simulink model "SMO_PLL_dq_model"  (R2024b)
settings: Solver=ode23  StartTime=0.0  StopTime=0.25  FixedStep=2e-7  RelTol=1e-3
InitFcn:
  | pn = 3;
  | Ld = 1.6e-3;
  | Lq = 1e-3;
  | Ls = Ld;
  | R = 0.011;
  | phi = 0.077;
  | J = 0.0008;
  | B = 0.000;
  | Ts = 1e-5;
undefined symbols (not defined in the file or in its folder): DiscIntNeverNeededParam
libraries: spsGroundLib x1, spsUniversalBridgeLib x1, spsPermanentMagnetSynchronousMachineLib x1, spsSVPWMGenerator2LevelLib x1, spsDCVoltageSourceLib x1, spspowerguiLib x1

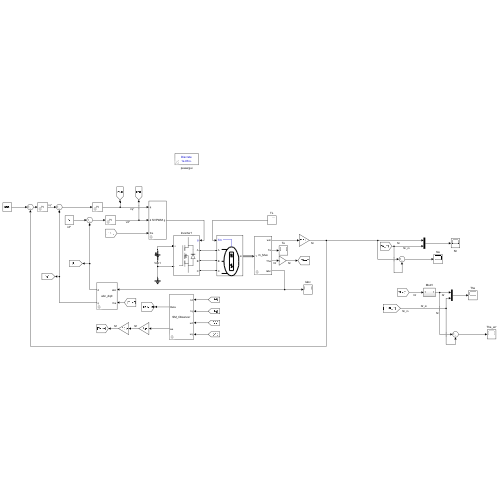
[thumbnail: Simulink's stored preview of the top-level diagram]
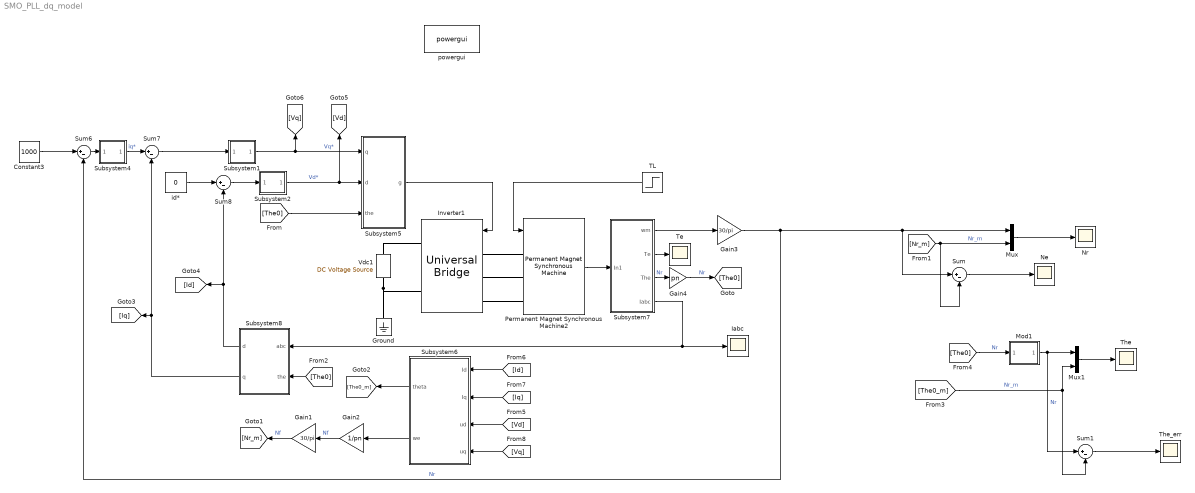
== system SMO_PLL_dq_model ==
  Constant3 : Constant  Value=1000
  Gain1 : Gain  Gain=30/pi
  Gain2 : Gain  Gain=1/pn
  Gain3 : Gain  Gain=30/pi
  Gain4 : Gain  Gain=pn
  Ground : spsGroundLib/Ground  LConnTagsString=a
  Iabc : Scope
  Inverter1 : spsUniversalBridgeLib/Universal Bridge  Arms=3  SnubberResistance=1e5  SnubberCapacitance=inf  Device=MOSFET / Diodes  Ron=1e-3  Lon=0  ForwardVoltages="[  0  0  ]"  ForwardVoltage=0  GTOparameters=[ 10e-6 , 20e-6 ]  IGBTparameters=[ 1e-6 , 2e-6 ]  Measurements=None  Measurements_2=None  converterType=Rectifier
  Mod1 : Subsystem
  Mux : Mux  Inputs=2
  Mux1 : Mux  Inputs=2
  Ne : Scope
  Nr : Scope
  Permanent Magnet Synchronous Machine2 : spsPermanentMagnetSynchronousMachineLib/Permanent Magnet Synchronous Machine  NbPhases=3  FluxDistribution=Sinusoidal  RotorType=Salient-pole  MechanicalLoad=Torque Tm  PresetModel=No  ShowDetailedParameters=on  MeasurementBus=off  Resistance=R  Inductance=8.5e-3  dqInductances=[Ld Lq]  La=0.000395  MachineConstant=Flux linkage established by magnets (V.s)  Flux=phi  VoltageCst=41.8988  TorqueCst=0.3465  Flat=120  Mechanical=[J B pn 0]  PolePairs=2  InitialConditions=[0,0, 0,0]  InitialConditions5ph=[0 0 0 0 0 0]  RefAngle=Aligned with phase A axis (original Park)  IterativeDiscreteModel=Trapezoidal non iterative  TsBlock=-1  TsPowergui=0
  Subsystem1 : Subsystem  mask{Ki=20000*R, Kp=20000*Lq, int_limit=[-161,161], out_limit=[-161,161], Ts=1/(10e3)}
      mask prompts: Ki "Ki : Integral"; Kp "Kp : Propotional"; int_limit "integral limit : [min, max]"; out_limit "output limit : [min, max]"; Ts "Ts : sample time"
  Subsystem2 : Subsystem  mask{Ki=10000*R, Kp=10000*Ld, int_limit=[-161,161], out_limit=[-161,161], Ts=1/(10e3)}
      mask prompts: Ki "Ki : Integral"; Kp "Kp : Propotional"; int_limit "integral limit : [min, max]"; out_limit "output limit : [min, max]"; Ts "Ts : sample time"
  Subsystem4 : Subsystem  mask{Ki=20, Kp=0.1, int_limit=[-200,200], out_limit=[-200,200], Ts=1/(5e3)}
      mask prompts: Ki "Ki : Integral"; Kp "Kp : Propotional"; int_limit "integral limit : [min, max]"; out_limit "output limit : [min, max]"; Ts "Ts : sample time"
  Subsystem5 : Subsystem  mask{Vdc=311}
  Subsystem6 : Subsystem  mask{Ts=1/(10e3), wc=300}
      mask prompts: Ts "Ts : sample time"; wc "wc : cross frequency (rad/s)"
  Subsystem7 : Subsystem
  Subsystem8 : Subsystem
  Sum{,1,6..8} (5 alike) : Sum  Inputs=|+-
  TL : Step  Time=0.1  After=10  SampleTime=0
  Te : Scope
  The : Scope
  The_err : Scope
  Vdc1 : spsDCVoltageSourceLib/DC Voltage Source  Amplitude=311  Measurements=None
  id* : Constant  Value=0
  powergui : spspowerguiLib/powergui  Priority=1  SimulationMode=Discrete  SampleTime=10e-7  frequency=60  Iterations=50  frequencyindice=0  Pbase=100e6  ErrMax=1e-4  UnitsV=kV  UnitsW=MW  buscounter=0  FunctionMessages=off  echomessages=off  EnableUseOfTLC=off  CurrentSourceSwitches=off  DisableSnubberDevices=off  DisableRonSwitches=off  DisableVfSwitches=off  DisplayEquations=off  AutomaticDiscreteSolvers=off  SolverType=Tustin/Backward Euler (TBE)  Interpol=off  ExternalGateDelay=off  methode=off  Ts=100  x0status=blocks  SPID=on  SwTol=0  HookPort=off  NonlinearTolerance=1e-4  nMaxIteration=100  ContinueOnMaxIteration=off  RestoreLinks=warning  ResistiveCurrentMeasurement=off  Frange=[0:2:500]  Ylog=off  Xlog=on  ShowGrid=off  save=off  variable=ZData  structure=0  ZoomFFT=off  StartTime=0.0  cycles=1  DisplayStyle=1  fundamental=60  FreqAxis=off  MaxFrequency=1000  frequencyindicesteady=1  RmsSteady=1  display=off
  wires:
  Sum7/1 -> Subsystem1/1(Input)
  Sum6/1 -> Subsystem4/1(Input)
  Subsystem4/1(output) -> Sum7/1  "iq*"
  Constant3/1 -> Sum6/1
  Subsystem5/1(g) -> Inverter1/1
  Subsystem7/1(wm) -> Gain3/1
  id*/1 -> Sum8/1
  Subsystem1/1(output) -> [Vq], Subsystem5/1(q)  "Vq*"
  Sum8/1 -> Subsystem2/1(Input)
  Subsystem2/1(output) -> Subsystem5/2(d), [Vd]  "Vd*"
  Subsystem8/2(q) -> [Iq], Sum7/2
  Subsystem7/2(Te) -> Te/1
  [The0] -> Subsystem5/3(the)
  Gain2/1 -> Gain1/1  "Nf"
  Subsystem6/2(we) -> Gain2/1
  Gain3/1 -> Sum6/2, Sum/1, Mux/1  "Nr"
  Mux/1 -> Nr/1
  Sum/1 -> Ne/1
  Subsystem7/3(The) -> Gain4/1  "Nr"
  TL/1 -> Permanent Magnet Synchronous Machine2/1
  Permanent Magnet Synchronous Machine2/1 -> Subsystem7/1(In1)
  [The0] -> Subsystem8/2(the)
  Gain4/1 -> [The0]  "Nr"
  Gain1/1 -> [Nr_m]  "Nf"
  [Nr_m] -> Sum/2, Mux/2  "Nr_m"
  Subsystem6/1(theta) -> [The0_m]
  [The0] -> Mod1/1(In1)  "Nr"
  Mux1/1 -> The/1
  [The0_m] -> Mux1/2, Sum1/2  "Nr_m"
  Mod1/1(Out1) -> Sum1/1, Mux1/1  "Nr"
  Sum1/1 -> The_err/1
  [Vq] -> Subsystem6/4(uq)
  [Vd] -> Subsystem6/3(ud)
  Subsystem8/1(d) -> [Id], Sum8/2
  [Id] -> Subsystem6/1(Id)
  [Iq] -> Subsystem6/2(Iq)
  Subsystem7/4(Iabc) -> Subsystem8/1(abc), Iabc/1
  connections:
  Vdc1/LConn1 -- Inverter1/RConn2 -- Ground/LConn1
  Vdc1/RConn1 -- Inverter1/RConn1
  Permanent Magnet Synchronous Machine2/LConn1 -- Inverter1/LConn1
  Inverter1/LConn3 -- Permanent Magnet Synchronous Machine2/LConn3
  Permanent Magnet Synchronous Machine2/LConn2 -- Inverter1/LConn2

== system SMO_PLL_dq_model/Mod1 ==
  In1 : Inport
  Constant1 : Constant  Value=2*pi
  Math Function : Math  Operator=mod  SignedPower=on
  Out1 : Outport
  wires:
  In1/1 -> Math Function/1
  Math Function/1 -> Out1/1
  Constant1/1 -> Math Function/2

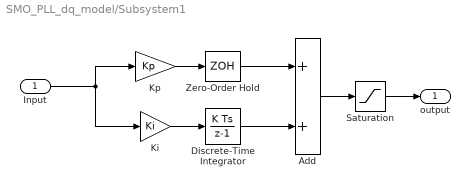
== system SMO_PLL_dq_model/Subsystem1 ==
  Input : Inport
  Add : Sum
  Discrete-Time Integrator : DiscreteIntegrator  SampleTime=Ts  LimitOutput=on  UpperSaturationLimit=int_limit(2)  LowerSaturationLimit=int_limit(1)  ICPrevOutput=DiscIntNeverNeededParam  ICPrevScaledInput=DiscIntNeverNeededParam
  Ki : Gain  Gain=Ki
  Kp : Gain  Gain=Kp
  Saturation : Saturate  UpperLimit=out_limit(2)  LowerLimit=out_limit(1)
  Zero-Order Hold : ZeroOrderHold  SampleTime=Ts
  output : Outport
  wires:
  Input/1 -> Ki/1, Kp/1
  Ki/1 -> Discrete-Time Integrator/1
  Discrete-Time Integrator/1 -> Add/2
  Add/1 -> Saturation/1
  Saturation/1 -> output/1
  Kp/1 -> Zero-Order Hold/1
  Zero-Order Hold/1 -> Add/1

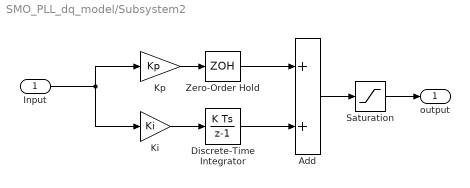
== system SMO_PLL_dq_model/Subsystem2 ==
  Input : Inport
  Add : Sum
  Discrete-Time Integrator : DiscreteIntegrator  SampleTime=Ts  LimitOutput=on  UpperSaturationLimit=int_limit(2)  LowerSaturationLimit=int_limit(1)  ICPrevOutput=DiscIntNeverNeededParam  ICPrevScaledInput=DiscIntNeverNeededParam
  Ki : Gain  Gain=Ki
  Kp : Gain  Gain=Kp
  Saturation : Saturate  UpperLimit=out_limit(2)  LowerLimit=out_limit(1)
  Zero-Order Hold : ZeroOrderHold  SampleTime=Ts
  output : Outport
  wires:
  Input/1 -> Ki/1, Kp/1
  Ki/1 -> Discrete-Time Integrator/1
  Discrete-Time Integrator/1 -> Add/2
  Add/1 -> Saturation/1
  Saturation/1 -> output/1
  Kp/1 -> Zero-Order Hold/1
  Zero-Order Hold/1 -> Add/1

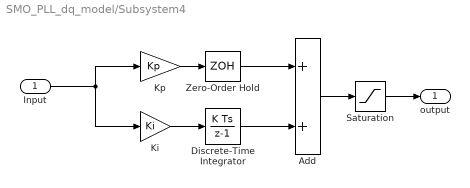
== system SMO_PLL_dq_model/Subsystem4 ==
  Input : Inport
  Add : Sum
  Discrete-Time Integrator : DiscreteIntegrator  SampleTime=Ts  LimitOutput=on  UpperSaturationLimit=int_limit(2)  LowerSaturationLimit=int_limit(1)  ICPrevOutput=DiscIntNeverNeededParam  ICPrevScaledInput=DiscIntNeverNeededParam
  Ki : Gain  Gain=Ki
  Kp : Gain  Gain=Kp
  Saturation : Saturate  UpperLimit=out_limit(2)  LowerLimit=out_limit(1)
  Zero-Order Hold : ZeroOrderHold  SampleTime=Ts
  output : Outport
  wires:
  Input/1 -> Ki/1, Kp/1
  Ki/1 -> Discrete-Time Integrator/1
  Discrete-Time Integrator/1 -> Add/2
  Add/1 -> Saturation/1
  Saturation/1 -> output/1
  Kp/1 -> Zero-Order Hold/1
  Zero-Order Hold/1 -> Add/1

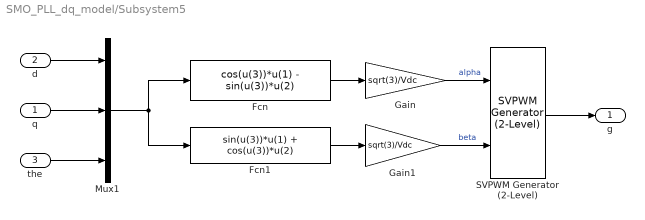
== system SMO_PLL_dq_model/Subsystem5 ==
  q : Inport
  d : Inport  Port=2
  the : Inport  Port=3
  Fcn : Fcn  Expr=cos(u(3))*u(1) - sin(u(3))*u(2)
  Fcn1 : Fcn  Expr=sin(u(3))*u(1) + cos(u(3))*u(2)
  Gain : Gain  Gain=sqrt(3)/Vdc
  Gain1 : Gain  Gain=sqrt(3)/Vdc
  Mux1 : Mux  Inputs=3
  SVPWM Generator (2-Level) : spsSVPWMGenerator2LevelLib/SVPWM Generator (2-Level)  InputType=alpha-beta components  SwitchingPattern=Pattern #1  Fc=10e3  ParUref=[0.8 -30 50]  Ts=0
  g : Outport
  wires:
  q/1 -> Mux1/2
  Fcn/1 -> Gain/1
  d/1 -> Mux1/1
  Fcn1/1 -> Gain1/1
  SVPWM Generator (2-Level)/1 -> g/1
  Mux1/1 -> Fcn/1, Fcn1/1
  the/1 -> Mux1/3
  Gain/1 -> SVPWM Generator (2-Level)/1  "alpha"
  Gain1/1 -> SVPWM Generator (2-Level)/2  "beta"

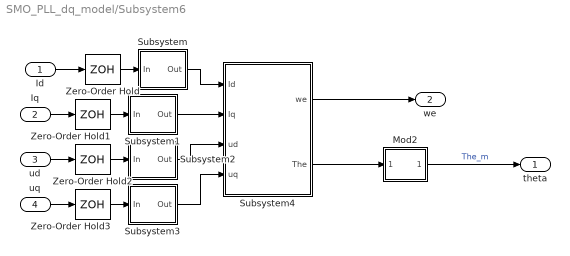
== system SMO_PLL_dq_model/Subsystem6 ==
  Id : Inport
  Iq : Inport  Port=2
  ud : Inport  Port=3
  uq : Inport  Port=4
  Mod2 : Subsystem
  Subsystem : Subsystem  mask{Ts=Ts, wc=wc}
      mask prompts: Ts "Ts ：sample time"; wc "wc : cross frequency (rad/s)"
  Subsystem1 : Subsystem  mask{Ts=Ts, wc=wc}
      mask prompts: Ts "Ts ：sample time"; wc "wc : cross frequency (rad/s)"
  Subsystem2 : Subsystem  mask{Ts=Ts, wc=wc}
      mask prompts: Ts "Ts ：sample time"; wc "wc : cross frequency (rad/s)"
  Subsystem3 : Subsystem  mask{Ts=Ts, wc=wc}
      mask prompts: Ts "Ts ：sample time"; wc "wc : cross frequency (rad/s)"
  Subsystem4 : Subsystem
  Zero-Order Hold{,1..3} (4 alike) : ZeroOrderHold  SampleTime=Ts
  theta : Outport
  we : Outport  Port=2
  wires:
  Subsystem4/1(we) -> we/1
  Subsystem4/2(The) -> Mod2/1(In1)
  Mod2/1(theta) -> theta/1  "The_m"
  Id/1 -> Zero-Order Hold/1
  Zero-Order Hold/1 -> Subsystem/1(In)
  Subsystem/1(Out) -> Subsystem4/1(Id)
  Subsystem1/1(Out) -> Subsystem4/2(Iq)
  Iq/1 -> Zero-Order Hold1/1
  Zero-Order Hold1/1 -> Subsystem1/1(In)
  Subsystem2/1(Out) -> Subsystem4/3(ud)
  ud/1 -> Zero-Order Hold2/1
  Zero-Order Hold2/1 -> Subsystem2/1(In)
  Subsystem3/1(Out) -> Subsystem4/4(uq)
  uq/1 -> Zero-Order Hold3/1
  Zero-Order Hold3/1 -> Subsystem3/1(In)

== system SMO_PLL_dq_model/Subsystem7 ==
  In1 : Inport
  Bus Selector1 : BusSelector  OutputSignals=Rotor speed wm (rad/s),Electromagnetic torque Te (N*m),Rotor angle thetam (rad),Stator current is_a (A),Stator current is_b (A),Stator current is_c (A)
  Mux : Mux  Inputs=3
  wm : Outport
  Te : Outport  Port=2
  The : Outport  Port=3
  Iabc : Outport  Port=4
  wires:
  In1/1 -> Bus Selector1/1
  Bus Selector1/1 -> wm/1  "<Rotor speed wm (rad/s)>"
  Bus Selector1/2 -> Te/1  "<Electromagnetic torque Te (N*m)>"
  Bus Selector1/3 -> The/1  "<Rotor angle thetam (rad)>"
  Bus Selector1/4 -> Mux/1  "<Stator current is_a (A)>"
  Bus Selector1/5 -> Mux/2  "<Stator current is_b (A)>"
  Bus Selector1/6 -> Mux/3  "<Stator current is_c (A)>"
  Mux/1 -> Iabc/1

== system SMO_PLL_dq_model/Subsystem8 ==
  abc : Inport
  the : Inport  Port=2
  Subsystem : Subsystem
  Subsystem5 : Subsystem
  d : Outport
  q : Outport  Port=2
  wires:
  Subsystem/1(d) -> d/1
  the/1 -> Subsystem/3(the)
  Subsystem5/2(beta) -> Subsystem/2(beta)
  Subsystem5/1(alpha) -> Subsystem/1(alpha)
  abc/1 -> Subsystem5/1(input)
  Subsystem/2(q) -> q/1

== system SMO_PLL_dq_model/Subsystem6/Mod2 ==
  In1 : Inport
  Constant1 : Constant  Value=2*pi
  Math Function : Math  Operator=mod  SignedPower=on
  theta : Outport
  wires:
  In1/1 -> Math Function/1
  Math Function/1 -> theta/1
  Constant1/1 -> Math Function/2

== system SMO_PLL_dq_model/Subsystem6/Subsystem ==
  In : Inport
  Delay : Delay  DelayLength=1  SampleTime=Ts
  Sum1 : Sum  Inputs=|++
  alpha : Gain  Gain=wc*Ts
  alpha1 : Gain  Gain=1-wc*Ts
  Out : Outport
  wires:
  alpha/1 -> Sum1/1
  Delay/1 -> alpha1/1
  In/1 -> alpha/1
  Sum1/1 -> Out/1, Delay/1
  alpha1/1 -> Sum1/2

== system SMO_PLL_dq_model/Subsystem6/Subsystem1 ==
  In : Inport
  Delay : Delay  DelayLength=1  SampleTime=Ts
  Sum1 : Sum  Inputs=|++
  alpha : Gain  Gain=wc*Ts
  alpha1 : Gain  Gain=1-wc*Ts
  Out : Outport
  wires:
  alpha/1 -> Sum1/1
  Delay/1 -> alpha1/1
  In/1 -> alpha/1
  Sum1/1 -> Out/1, Delay/1
  alpha1/1 -> Sum1/2

== system SMO_PLL_dq_model/Subsystem6/Subsystem2 ==
  In : Inport
  Delay : Delay  DelayLength=1  SampleTime=Ts
  Sum1 : Sum  Inputs=|++
  alpha : Gain  Gain=wc*Ts
  alpha1 : Gain  Gain=1-wc*Ts
  Out : Outport
  wires:
  alpha/1 -> Sum1/1
  Delay/1 -> alpha1/1
  In/1 -> alpha/1
  Sum1/1 -> Out/1, Delay/1
  alpha1/1 -> Sum1/2

== system SMO_PLL_dq_model/Subsystem6/Subsystem3 ==
  In : Inport
  Delay : Delay  DelayLength=1  SampleTime=Ts
  Sum1 : Sum  Inputs=|++
  alpha : Gain  Gain=wc*Ts
  alpha1 : Gain  Gain=1-wc*Ts
  Out : Outport
  wires:
  alpha/1 -> Sum1/1
  Delay/1 -> alpha1/1
  In/1 -> alpha/1
  Sum1/1 -> Out/1, Delay/1
  alpha1/1 -> Sum1/2

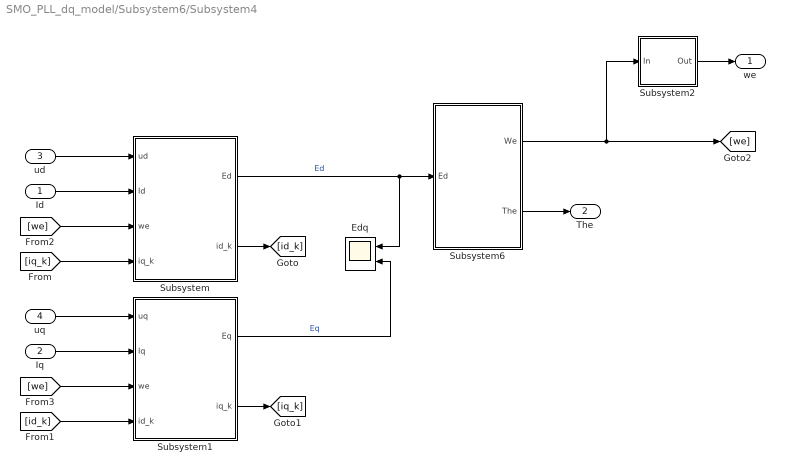
== system SMO_PLL_dq_model/Subsystem6/Subsystem4 ==
  Id : Inport
  Iq : Inport  Port=2
  ud : Inport  Port=3
  uq : Inport  Port=4
  Edq : Scope  NumInputPorts=2
  Subsystem : Subsystem
  Subsystem1 : Subsystem
  Subsystem2 : Subsystem  mask{Ts=Ts, wc=wc/3}
      mask prompts: Ts "Ts ：sample time"; wc "wc : cross frequency (rad/s)"
  Subsystem6 : Subsystem
  we : Outport
  The : Outport  Port=2
  wires:
  ud/1 -> Subsystem/1(ud)
  Id/1 -> Subsystem/2(Id)
  uq/1 -> Subsystem1/1(uq)
  Iq/1 -> Subsystem1/2(Iq)
  Subsystem/1(Ed) -> Subsystem6/1(Ed), Edq/1  "Ed"
  Subsystem1/1(Eq) -> Edq/2  "Eq"
  Subsystem/2(id_k) -> [id_k]
  Subsystem1/2(iq_k) -> [iq_k]
  [iq_k] -> Subsystem/4(iq_k)
  [id_k] -> Subsystem1/4(id_k)
  [we] -> Subsystem/3(we)
  [we] -> Subsystem1/3(we)
  Subsystem6/1(We) -> Subsystem2/1(In), [we]
  Subsystem6/2(The) -> The/1
  Subsystem2/1(Out) -> we/1

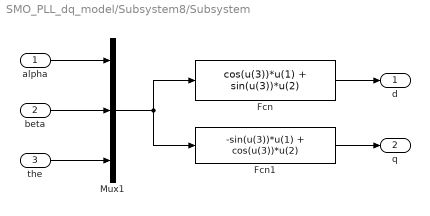
== system SMO_PLL_dq_model/Subsystem8/Subsystem ==
  alpha : Inport
  beta : Inport  Port=2
  the : Inport  Port=3
  Fcn : Fcn  Expr=cos(u(3))*u(1) + sin(u(3))*u(2)
  Fcn1 : Fcn  Expr=-sin(u(3))*u(1) + cos(u(3))*u(2)
  Mux1 : Mux  Inputs=3
  d : Outport
  q : Outport  Port=2
  wires:
  Fcn/1 -> d/1
  Mux1/1 -> Fcn/1, Fcn1/1
  the/1 -> Mux1/3
  beta/1 -> Mux1/2
  Fcn1/1 -> q/1
  alpha/1 -> Mux1/1

== system SMO_PLL_dq_model/Subsystem8/Subsystem5 ==
  input : Inport
  Demux : Demux  Outputs=3
  Subsystem : Subsystem
  alpha : Outport
  beta : Outport  Port=2
  wires:
  input/1 -> Demux/1
  Demux/1 -> Subsystem/1(a)
  Demux/2 -> Subsystem/2(b)
  Demux/3 -> Subsystem/3(c)
  Subsystem/1(alpha) -> alpha/1
  Subsystem/2(beta) -> beta/1

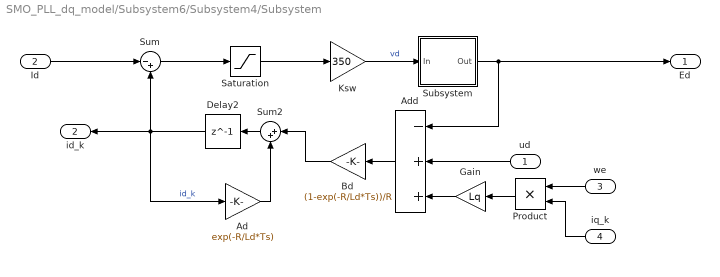
== system SMO_PLL_dq_model/Subsystem6/Subsystem4/Subsystem ==
  ud : Inport
  Id : Inport  Port=2
  we : Inport  Port=3
  iq_k : Inport  Port=4
  Ad : Gain  Gain=exp(-R/Ld*Ts)
  Add : Sum  Inputs=-++
  Bd : Gain  Gain=(1-exp(-R/Ld*Ts))/R
  Delay2 : Delay  DelayLength=1  SampleTime=Ts
  Gain : Gain  Gain=Lq
  Ksw : Gain  Gain=350
  Product : Product
  Saturation : Saturate  UpperLimit=2  LowerLimit=-2
  Subsystem : Subsystem  mask{Ts=Ts, wc=wc}
      mask prompts: Ts "Ts ：sample time"; wc "wc : cross frequency (rad/s)"
  Sum : Sum  Inputs=|-+
  Sum2 : Sum  Inputs=|++
  Ed : Outport
  id_k : Outport  Port=2
  wires:
  Ksw/1 -> Subsystem/1(In)  "vd"
  Sum/1 -> Saturation/1
  Saturation/1 -> Ksw/1
  ud/1 -> Add/2
  Add/1 -> Bd/1
  Bd/1 -> Sum2/1
  Id/1 -> Sum/1
  Ad/1 -> Sum2/2
  Delay2/1 -> id_k/1, Ad/1, Sum/2  "id_k"
  Sum2/1 -> Delay2/1
  Subsystem/1(Out) -> Add/1, Ed/1
  Gain/1 -> Add/3
  Product/1 -> Gain/1
  we/1 -> Product/1
  iq_k/1 -> Product/2

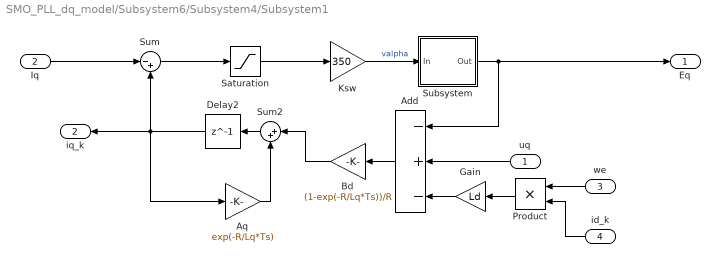
== system SMO_PLL_dq_model/Subsystem6/Subsystem4/Subsystem1 ==
  uq : Inport
  Iq : Inport  Port=2
  we : Inport  Port=3
  id_k : Inport  Port=4
  Add : Sum  Inputs=-+-
  Aq : Gain  Gain=exp(-R/Lq*Ts)
  Bd : Gain  Gain=(1-exp(-R/Lq*Ts))/R
  Delay2 : Delay  DelayLength=1  SampleTime=Ts
  Gain : Gain  Gain=Ld
  Ksw : Gain  Gain=350
  Product : Product
  Saturation : Saturate  UpperLimit=2  LowerLimit=-2
  Subsystem : Subsystem  mask{Ts=Ts, wc=wc}
      mask prompts: Ts "Ts ：sample time"; wc "wc : cross frequency (rad/s)"
  Sum : Sum  Inputs=|-+
  Sum2 : Sum  Inputs=|++
  Eq : Outport
  iq_k : Outport  Port=2
  wires:
  Ksw/1 -> Subsystem/1(In)  "valpha"
  Sum/1 -> Saturation/1
  Saturation/1 -> Ksw/1
  uq/1 -> Add/2
  Add/1 -> Bd/1
  Bd/1 -> Sum2/1
  Iq/1 -> Sum/1
  Aq/1 -> Sum2/2
  Delay2/1 -> iq_k/1, Aq/1, Sum/2
  Sum2/1 -> Delay2/1
  Subsystem/1(Out) -> Add/1, Eq/1
  Gain/1 -> Add/3
  Product/1 -> Gain/1
  we/1 -> Product/1
  id_k/1 -> Product/2

== system SMO_PLL_dq_model/Subsystem6/Subsystem4/Subsystem2 ==
  In : Inport
  Delay : Delay  DelayLength=1  SampleTime=Ts
  Sum1 : Sum  Inputs=|++
  alpha : Gain  Gain=wc*Ts
  alpha1 : Gain  Gain=1-wc*Ts
  Out : Outport
  wires:
  alpha/1 -> Sum1/1
  Delay/1 -> alpha1/1
  In/1 -> alpha/1
  Sum1/1 -> Out/1, Delay/1
  alpha1/1 -> Sum1/2

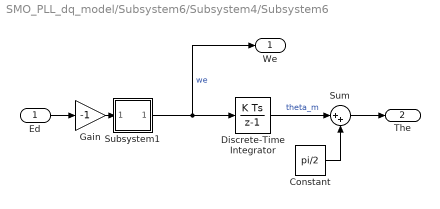
== system SMO_PLL_dq_model/Subsystem6/Subsystem4/Subsystem6 ==
  Ed : Inport
  Constant : Constant  Value=pi/2
  Discrete-Time Integrator : DiscreteIntegrator  SampleTime=Ts  ICPrevOutput=DiscIntNeverNeededParam  ICPrevScaledInput=DiscIntNeverNeededParam
  Gain : Gain  Gain=-1
  Subsystem1 : Subsystem  mask{Ki=6000, Kp=30, int_limit=[-1000,1000], out_limit=[-1000,1000], Ts=1/(10e3)}
      mask prompts: Ki "Ki : Integral"; Kp "Kp : Propotional"; int_limit "integral limit : [min, max]"; out_limit "output limit : [min, max]"; Ts "Ts : sample time"
  Sum : Sum  Inputs=|++
  We : Outport
  The : Outport  Port=2
  wires:
  Subsystem1/1(output) -> We/1, Discrete-Time Integrator/1  "we"
  Gain/1 -> Subsystem1/1(Input)
  Discrete-Time Integrator/1 -> Sum/1  "theta_m"
  Sum/1 -> The/1
  Constant/1 -> Sum/2
  Ed/1 -> Gain/1

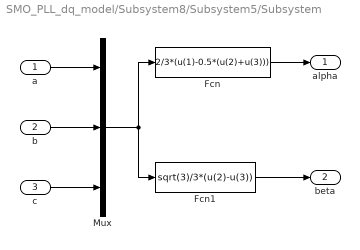
== system SMO_PLL_dq_model/Subsystem8/Subsystem5/Subsystem ==
  a : Inport
  b : Inport  Port=2
  c : Inport  Port=3
  Fcn : Fcn  Expr=2/3*(u(1)-0.5*(u(2)+u(3)))
  Fcn1 : Fcn  Expr=sqrt(3)/3*(u(2)-u(3))
  Mux : Mux  Inputs=3
  alpha : Outport
  beta : Outport  Port=2
  wires:
  a/1 -> Mux/1
  b/1 -> Mux/2
  c/1 -> Mux/3
  Mux/1 -> Fcn/1, Fcn1/1
  Fcn/1 -> alpha/1
  Fcn1/1 -> beta/1

== system SMO_PLL_dq_model/Subsystem6/Subsystem4/Subsystem/Subsystem ==
  In : Inport
  Delay : Delay  DelayLength=1  SampleTime=Ts
  Sum1 : Sum  Inputs=|++
  alpha : Gain  Gain=wc*Ts
  alpha1 : Gain  Gain=1-wc*Ts
  Out : Outport
  wires:
  alpha/1 -> Sum1/1
  Delay/1 -> alpha1/1
  In/1 -> alpha/1
  Sum1/1 -> Out/1, Delay/1
  alpha1/1 -> Sum1/2

== system SMO_PLL_dq_model/Subsystem6/Subsystem4/Subsystem1/Subsystem ==
  In : Inport
  Delay : Delay  DelayLength=1  SampleTime=Ts
  Sum1 : Sum  Inputs=|++
  alpha : Gain  Gain=wc*Ts
  alpha1 : Gain  Gain=1-wc*Ts
  Out : Outport
  wires:
  alpha/1 -> Sum1/1
  Delay/1 -> alpha1/1
  In/1 -> alpha/1
  Sum1/1 -> Out/1, Delay/1
  alpha1/1 -> Sum1/2

== system SMO_PLL_dq_model/Subsystem6/Subsystem4/Subsystem6/Subsystem1 ==
  Input : Inport
  Add : Sum
  Discrete-Time Integrator : DiscreteIntegrator  SampleTime=Ts  LimitOutput=on  UpperSaturationLimit=int_limit(2)  LowerSaturationLimit=int_limit(1)  ICPrevOutput=DiscIntNeverNeededParam  ICPrevScaledInput=DiscIntNeverNeededParam
  Ki : Gain  Gain=Ki
  Kp : Gain  Gain=Kp
  Saturation : Saturate  UpperLimit=out_limit(2)  LowerLimit=out_limit(1)
  Zero-Order Hold : ZeroOrderHold  SampleTime=Ts
  output : Outport
  wires:
  Input/1 -> Ki/1, Kp/1
  Ki/1 -> Discrete-Time Integrator/1
  Discrete-Time Integrator/1 -> Add/2
  Add/1 -> Saturation/1
  Saturation/1 -> output/1
  Kp/1 -> Zero-Order Hold/1
  Zero-Order Hold/1 -> Add/1
